simulink model "W3Q2"  (R2020a)
settings: Solver=VariableStepAuto  StartTime=0.0  StopTime=10.0  RelTol=1e-3
settings Model: Creator=Vinayak  LastModifiedBy=Vinayak

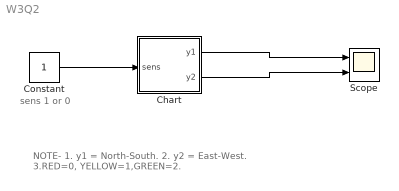
== system W3Q2 ==
  note: sens 1 or 0
  note: NOTE-
      |
      | 1. y1 = North-South.
      | 2. y2 = East-West.
      | 3.RED=0, YELLOW=1,GREEN=2.
  Chart : Stateflow chart  TreatAsAtomicUnit=on
  Constant : Constant
  Scope : Scope  NumInputPorts=2
  wires:
  Chart/2(y2) -> Scope/2
  Chart/1(y1) -> Scope/1
  Constant/1 -> Chart/1(sens)

== stateflow chart W3Q2/Chart ==
  state stop
    y1=RED;
    y2=GREEN;
  state stopfortraff
    y1=RED;
    y2=GREEN;
  state stoptogo
    y1=RED;
    y2=YELLOW;
  state go
    y1=GREEN;
    y2=RED;
  state gotostop
    y1=YELLOW;
    y2=RED;
  (default) -> stop
  stop -> stopfortraff : after(20,tick)
  stopfortraff -> stoptogo : [sens==1]
  gotostop -> stop : after(3,tick)
  stoptogo -> go : after(3,tick)
  go -> gotostop : after(10,tick)
  data: GREEN local =2; YELLOW local =1; RED local =0; y1 output; y2 output; sens input
